simulink model "HeightModel_mrft"  (R2012b)
settings: Solver=ode1  SolverMode=SingleTasking  StartTime=0.0  StopTime=t_final  FixedStep=time_step  RelTol=1e-3
values from neighbouring files (symbols this model uses):
  beta_mrft = -0.8    [main.m]    (also in main_normalized.m = -0.73)
  bias_acc = (2*rand()-1) * 7    [main.m]    (also in mesh_generation.m = 0; mesh_generation_normalized.m = 0)
  gain = gain_grid(i)    [main.m]    (also in main_normalized.m = final_points_normalized(1,5); mesh_generation.m = gain_mesh(i2_gain); mesh_generation_normalized.m = 1)
  h_mrft = 0.1    [main.m]    (also in main_normalized.m)
  init_val = 0    [main.m]    (also in main_normalized.m = 0.001; mesh_generation.m; mesh_generation_normalized.m)
  ref_val = 1    [main.m]    (also in main_normalized.m = 0; mesh_generation.m; mesh_generation_normalized.m)
  sigma_h = 0*0.001^2    (= 0)    [main.m]    (also in main_normalized.m = amplitude*0.05; mesh_generation.m; mesh_generation_normalized.m)
  T_body = T_body_grid(i)    [main.m]    (also in main_normalized.m = 0.2; mesh_generation.m = T_body_mesh(i2_T_body); mesh_generation_normalized.m = ratio_2_mesh(i2_ratio_2) * tau)
  T_prop = T_prop_grid(i)    [main.m]    (also in main_normalized.m = 0.015; mesh_generation.m = T_prop_mesh(i2_T_prop); mesh_generation_normalized.m = ratio_1_mesh(i2_ratio_1) * tau)
  tau = tau_grid(i)    [main.m]    (also in main_normalized.m = (0.1-0.001) * rand + 0.001; mesh_generation.m = tau_mesh(i2_tau); mesh_generation_normalized.m = 0.01)
  time_step = 0.001    [main.m]    (also in main_normalized.m = 0.0001; mesh_generation.m = min([tau, 0.1*min([T_body, T_prop])]); mesh_generation_normalized.m = min([tau, 0.1*min([T_body, T_prop])]))
libraries: simulink x1
settings Model: Creator=mchehadeh  LastModifiedBy=aaa_b
settings OptimizationCC: BlockReduction=off  BooleanDataType=off
settings DebuggingCC: SaveWithParameterizedLinksMsg=none  SignalResolutionControl=TryResolveAllWithWarning  SolverPrmCheckMsg=none  MultiTaskDSMMsg=warning  MultiTaskCondExecSysMsg=none  StrictBusMsg=None
settings HardwareCC: TargetUnknown=on
settings RTWCC: IncludeERTFirstTime=on

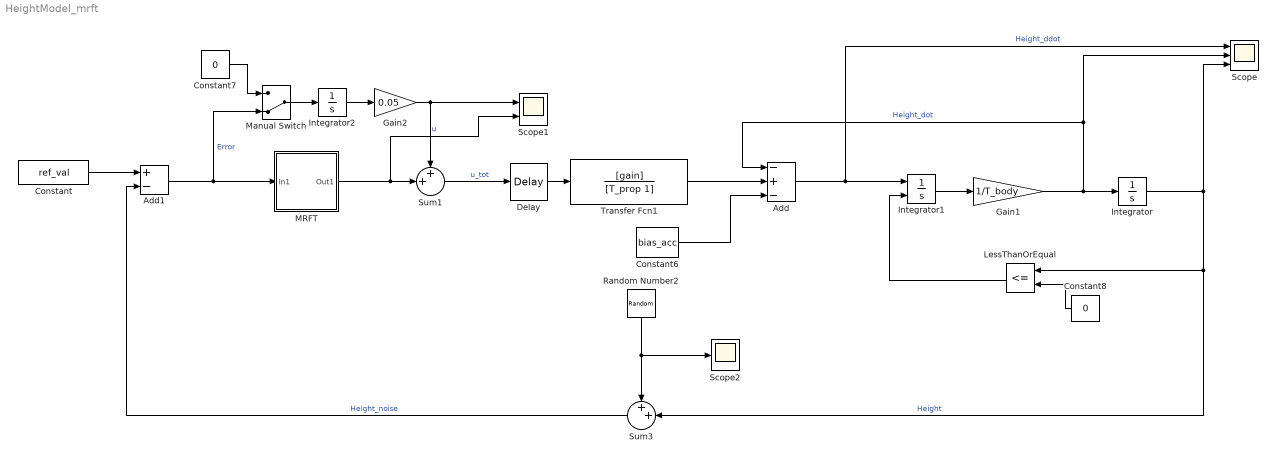
== system HeightModel_mrft ==
  Add : Sum  Inputs=-+-
  Add1 : Sum  Inputs=+-
  Constant : Constant  Value=ref_val
  Constant6 : Constant  Value=bias_acc
  Constant7 : Constant  Value=0
  Constant8 : Constant  Value=0
  "Delay " : TransportDelay  DelayTime=tau  InitialOutput=init_val
  Gain1 : Gain  Gain=1/T_body
  Gain2 : Gain  Gain=0.05
  Integrator : Integrator  InitialCondition=init_val  LimitOutput=on  LowerSaturationLimit=0
  Integrator1 : Integrator  ExternalReset=rising
  Integrator2 : Integrator
  LessThanOrEqual : RelationalOperator  Operator=<=  OutDataTypeStr=boolean
  MRFT : Subsystem
  Manual Switch : ManualSwitch  CurrentSetting=0
  Random Number2 : RandomNumber  Variance=sigma_h  SampleTime=time_step
  Scope : Scope  NumInputPorts=3
      settings: YMin=-5~-5~-5  YMax=5~5~5
  Scope1 : Scope  NumInputPorts=2
  Scope2 : Scope
  Sum1 : Sum  Inputs=++|
  Sum3 : Sum  Inputs=++|
  Transfer Fcn1 : TransferFcn  Numerator=[gain]  Denominator=[T_prop 1]
  wires:
  Gain1/1 -> Scope/2, Add/1, Integrator/1  "Height_dot"
  Integrator/1 -> Scope/3, LessThanOrEqual/1, Sum3/2  "Height"
  Constant/1 -> Add1/1
  Sum3/1 -> Add1/2  "Height_noise"
  Random Number2/1 -> Scope2/1, Sum3/1
  Add/1 -> Scope/1, Integrator1/1  "Height_ddot"
  Add1/1 -> MRFT/1(In1), Manual Switch/2  "Error"
  Integrator2/1 -> Gain2/1
  Constant6/1 -> Add/3
  Gain2/1 -> Scope1/1, Sum1/1
  Constant7/1 -> Manual Switch/1
  Manual Switch/1 -> Integrator2/1
  "Delay "/1 -> Transfer Fcn1/1
  Sum1/1 -> "Delay "/1  "u_tot"
  MRFT/1(Out1) -> Sum1/2, Scope1/2  "u"
  Constant8/1 -> LessThanOrEqual/2
  LessThanOrEqual/1 -> Integrator1/2
  Transfer Fcn1/1 -> Add/2
  Integrator1/1 -> Gain1/1

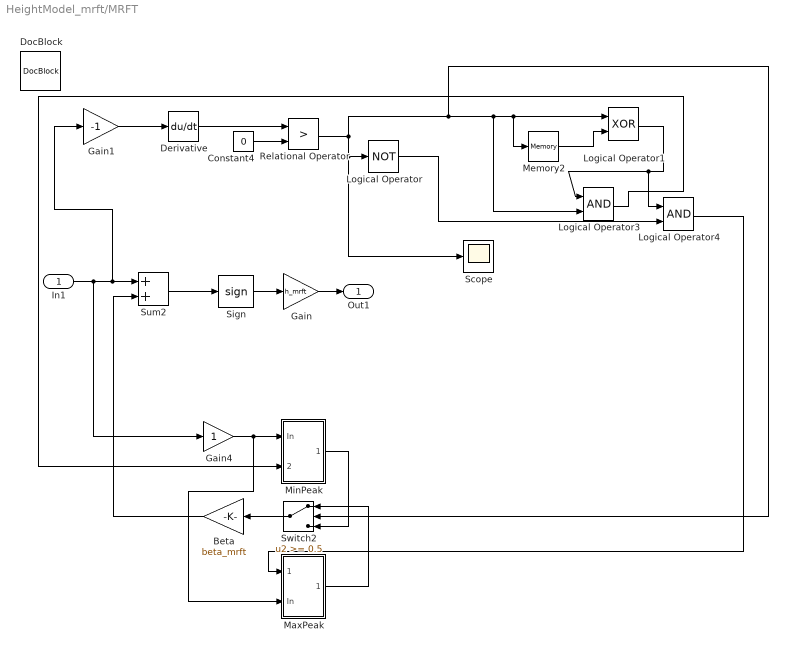
== system HeightModel_mrft/MRFT ==
  In1 : Inport
  Beta : Gain  Gain=beta_mrft  SaturateOnIntegerOverflow=on  OutDataTypeStr=Inherit: Same as input  ParamDataTypeStr=Inherit: Same as input
  Constant4 : Constant  Value=0
  Derivative : Derivative  CoefficientInTFapproximation=0.0002
  DocBlock : simulink/Model-Wide Utilities/DocBlock  DocumentType=Text
  Gain : Gain  Gain=h_mrft  SaturateOnIntegerOverflow=on  OutDataTypeStr=Inherit: Same as input  ParamDataTypeStr=Inherit: Same as input
  Gain1 : Gain  Gain=-1  SaturateOnIntegerOverflow=on  OutDataTypeStr=Inherit: Same as input  ParamDataTypeStr=Inherit: Same as input
  Gain4 : Gain  SaturateOnIntegerOverflow=on  OutDataTypeStr=Inherit: Same as input  ParamDataTypeStr=Inherit: Same as input
  Logical Operator : Logic  Operator=NOT  Inputs=1
  Logical Operator1 : Logic  Operator=XOR
  Logical Operator3 : Logic
  Logical Operator4 : Logic
  MaxPeak : Subsystem
  Memory2 : Memory
  MinPeak : Subsystem
  Relational Operator : RelationalOperator  Operator=>  InputSameDT=on
  Scope : Scope
  Sign : Signum
  Sum2 : Sum  SaturateOnIntegerOverflow=on  InputSameDT=on  OutDataTypeStr=Inherit: Same as first input
  Switch2 : Switch  Threshold=0.5  SaturateOnIntegerOverflow=on  InputSameDT=on
  Out1 : Outport
  wires:
  Memory2/1 -> Logical Operator1/2
  Switch2/1 -> Beta/1
  Logical Operator1/1 -> Logical Operator4/1, Logical Operator3/1
  Logical Operator4/1 -> MaxPeak/1(Cntrl)
  Constant4/1 -> Relational Operator/2
  Relational Operator/1 -> Scope/1, Logical Operator/1, Logical Operator1/1, Memory2/1, Logical Operator3/2, Switch2/2
  Logical Operator3/1 -> MinPeak/2(Cntrl)
  Logical Operator/1 -> Logical Operator4/2
  Sign/1 -> Gain/1
  Gain4/1 -> MinPeak/1(In), MaxPeak/2(In)
  Sum2/1 -> Sign/1
  Beta/1 -> Sum2/2
  MaxPeak/1(Out) -> Switch2/1
  MinPeak/1(Out) -> Switch2/3
  Derivative/1 -> Relational Operator/1
  Gain/1 -> Out1/1
  In1/1 -> Gain4/1, Gain1/1, Sum2/1
  Gain1/1 -> Derivative/1

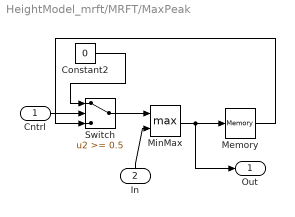
== system HeightModel_mrft/MRFT/MaxPeak ==
  Cntrl : Inport
  In : Inport  Port=2
  Constant2 : Constant  Value=0
  Memory : Memory
  MinMax : MinMax  Function=max  Inputs=2  SaturateOnIntegerOverflow=on  InputSameDT=on
  Switch : Switch  Threshold=0.5  SaturateOnIntegerOverflow=on  InputSameDT=on
  Out : Outport
  wires:
  MinMax/1 -> Memory/1, Out/1
  Switch/1 -> MinMax/1
  Constant2/1 -> Switch/1
  Memory/1 -> Switch/3
  In/1 -> MinMax/2
  Cntrl/1 -> Switch/2

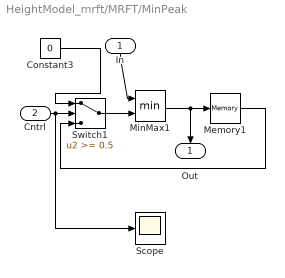
== system HeightModel_mrft/MRFT/MinPeak ==
  In : Inport
  Cntrl : Inport  Port=2
  Constant3 : Constant  Value=0
  Memory1 : Memory
  MinMax1 : MinMax  Inputs=2  SaturateOnIntegerOverflow=on  InputSameDT=on
  Scope : Scope
  Switch1 : Switch  Threshold=0.5  SaturateOnIntegerOverflow=on  InputSameDT=on
  Out : Outport
  wires:
  MinMax1/1 -> Memory1/1, Out/1
  Switch1/1 -> MinMax1/2
  Memory1/1 -> Switch1/3
  Constant3/1 -> Switch1/1
  In/1 -> MinMax1/1
  Cntrl/1 -> Switch1/2, Scope/1
